simulink model "noise_suppression"  (R2020b)
settings: Solver=FixedStepDiscrete  StartTime=0.0  StopTime=stopTime  RelTol=1e-3
InitFcn:
  | initCallback
StopFcn:
  | stopCallback
values from neighbouring files (symbols this model uses):
  mp = sm_init_avalon_signals(mp)    [sm_callback_init.m]
undefined symbols (not defined in the file or in its folder): config
libraries: hdlsllib x1
settings Model: Creator=Ross  LastModifiedBy=tyler
settings SolverCC: AutoInsertRateTranBlk=on
settings DataIOCC: ReturnWorkspaceOutputs=off
settings OptimizationCC: BlockReduction=off  ConditionallyExecuteInputs=off  DefaultParameterBehavior=Inlined
settings DebuggingCC: SignalInfNanChecking=error  SignalRangeChecking=warning  ReadBeforeWriteMsg=DisableAll  WriteAfterWriteMsg=DisableAll  WriteAfterReadMsg=DisableAll  AlgebraicLoopMsg=error  MultiTaskDSMMsg=none  SingleTaskRateTransMsg=error  ParameterUnderflowMsg=warning  UnderSpecifiedDataTypeMsg=error  PregeneratedLibrarySubsystemCodeDiagnostic=none  ArithmeticOperatorsInVariantConditions=warning
settings HardwareCC: ProdBitPerPointer=32  ProdBitPerSizeT=32  ProdBitPerPtrDiffT=32  ProdLargestAtomicFloat=None  ProdIntDivRoundTo=Undefined  ProdEndianess=Unspecified  ProdWordSize=32  ProdHWDeviceType=ASIC/FPGA->ASIC/FPGA  TargetBitPerPointer=64  TargetBitPerSizeT=64  TargetBitPerPtrDiffT=64  TargetLongLongMode=on  TargetIntDivRoundTo=Zero  TargetEndianess=LittleEndian  TargetWordSize=64  TargetHWDeviceType=Custom Processor->MATLAB Host Computer  ProdEqTarget=off
settings ModelReferenceCC: UpdateModelReferenceTargets=IfOutOfDate
settings SFSimCC: SFSimEcho=off  SimUseLocalCustomCode=off  CustomCodeUndefinedFunction=UseInterfaceOnly
settings RTWCC: RTWUseLocalCustomCode=off

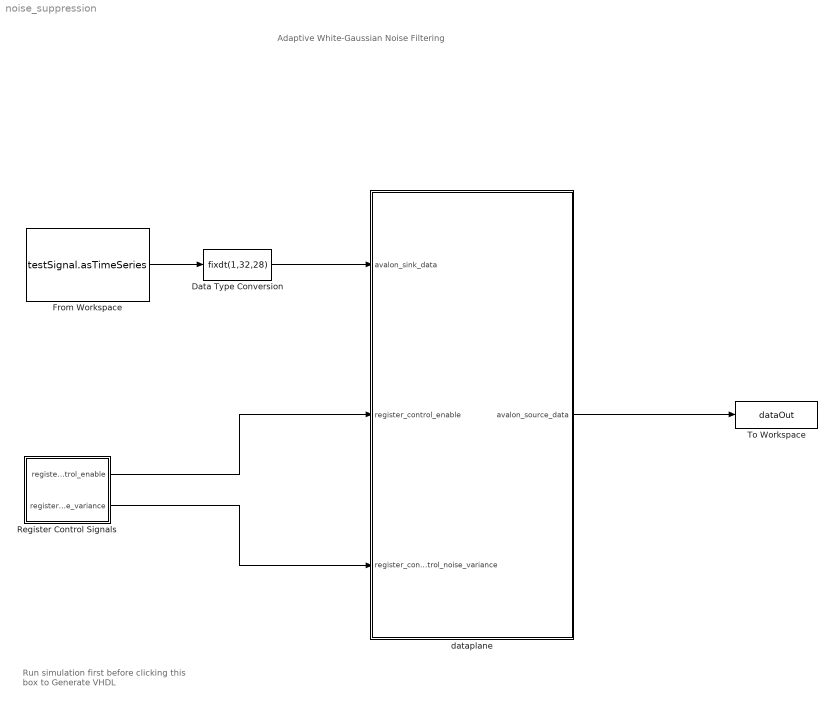
== system noise_suppression ==
  note: Adaptive White-Gaussian Noise Filtering
  note: Run simulation first
      | before clicking this box to
      | Generate VHDL
  Data Type Conversion : DataTypeConversion  OutDataTypeStr=fixdt(1,32,28)
  From Workspace : FromWorkspace  VariableName=testSignal.asTimeSeries  OutDataTypeStr=double  SampleTime=1 / config.system.sampleClockFrequency  Interpolate=off  OutputAfterFinalValue=Setting to zero
  Register Control Signals : Subsystem
  To Workspace : ToWorkspace  VariableName=dataOut  SaveFormat=Timeseries  SampleTime=-1
      settings: Save2DSignal=2-D array (concatenate along first dimension)
  dataplane : Subsystem  TreatAsAtomicUnit=on
  wires:
  dataplane/1(avalon_source_data) -> To Workspace/1
  From Workspace/1 -> Data Type Conversion/1
  Data Type Conversion/1 -> dataplane/1(avalon_sink_data)
  Register Control Signals/1(register_control_enable) -> dataplane/2(register_control_enable)
  Register Control Signals/2(register_control_noise_variance) -> dataplane/3(register_control_noise_variance)

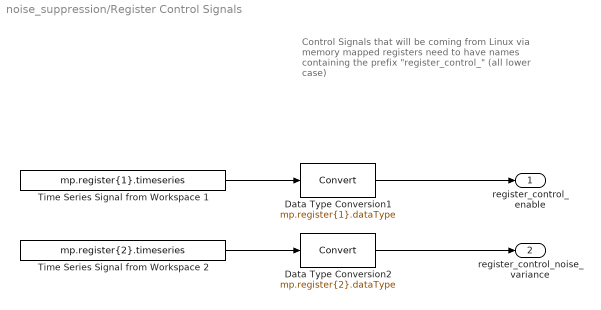
== system noise_suppression/Register Control Signals ==
  note: Control Signals that will be coming from Linux via
      | memory mapped registers need to have names
      | containing the prefix "register_control_"
      | (all lower case)
  Data Type Conversion1 : DataTypeConversion  OutDataTypeStr=mp.register{1}.dataType
  Data Type Conversion2 : DataTypeConversion  OutDataTypeStr=mp.register{2}.dataType
  Time Series Signal from Workspace 1 : FromWorkspace  VariableName=mp.register{1}.timeseries  OutDataTypeStr=double  SampleTime=1 / config.system.sampleClockFrequency
  Time Series Signal from Workspace 2 : FromWorkspace  VariableName=mp.register{2}.timeseries  OutDataTypeStr=double  SampleTime=1 / config.system.sampleClockFrequency
  register_control_enable : Outport  VectorParamsAs1DForOutWhenUnconnected=off
  register_control_noise_variance : Outport  Port=2  VectorParamsAs1DForOutWhenUnconnected=off
  wires:
  Time Series Signal from Workspace 1/1 -> Data Type Conversion1/1
  Data Type Conversion1/1 -> register_control_enable/1
  Time Series Signal from Workspace 2/1 -> Data Type Conversion2/1
  Data Type Conversion2/1 -> register_control_noise_variance/1

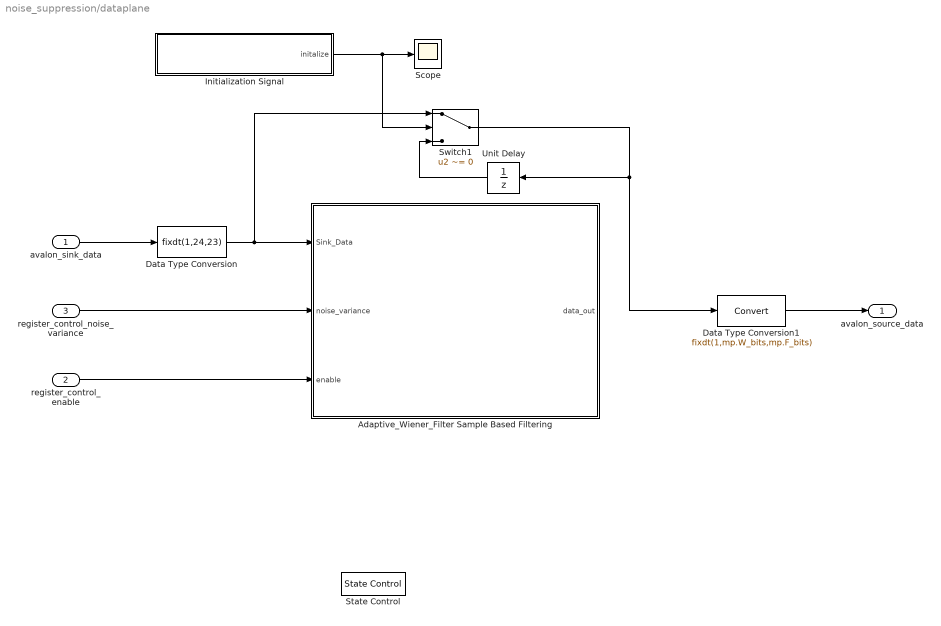
== system noise_suppression/dataplane ==
  avalon_sink_data : Inport
  register_control_enable : Inport  Port=2
  register_control_noise_variance : Inport  Port=3
  Adaptive_Wiener_Filter Sample Based Filtering : Subsystem
  Data Type Conversion : DataTypeConversion  OutDataTypeStr=fixdt(1,24,23)
  Data Type Conversion1 : DataTypeConversion  OutDataTypeStr=fixdt(1,mp.W_bits,mp.F_bits)
  Initialization Signal : Subsystem
  Scope : Scope
  State Control : StateControl  StateControl=Synchronous
  Switch1 : Switch  Criteria=u2 ~= 0  OutDataTypeStr=fixdt(1,24,23)
  Unit Delay : UnitDelay  SampleTime=-1  HasFrameUpgradeWarning=on
  avalon_source_data : Outport  VectorParamsAs1DForOutWhenUnconnected=off
  wires:
  avalon_sink_data/1 -> Data Type Conversion/1
  register_control_enable/1 -> Adaptive_Wiener_Filter Sample Based Filtering/3(enable)
  register_control_noise_variance/1 -> Adaptive_Wiener_Filter Sample Based Filtering/2(noise_variance)
  Data Type Conversion/1 -> Switch1/1, Adaptive_Wiener_Filter Sample Based Filtering/1(Sink_Data)
  Unit Delay/1 -> Switch1/3
  Switch1/1 -> Data Type Conversion1/1, Unit Delay/1
  Data Type Conversion1/1 -> avalon_source_data/1
  Initialization Signal/1(initalize) -> Scope/1, Switch1/2

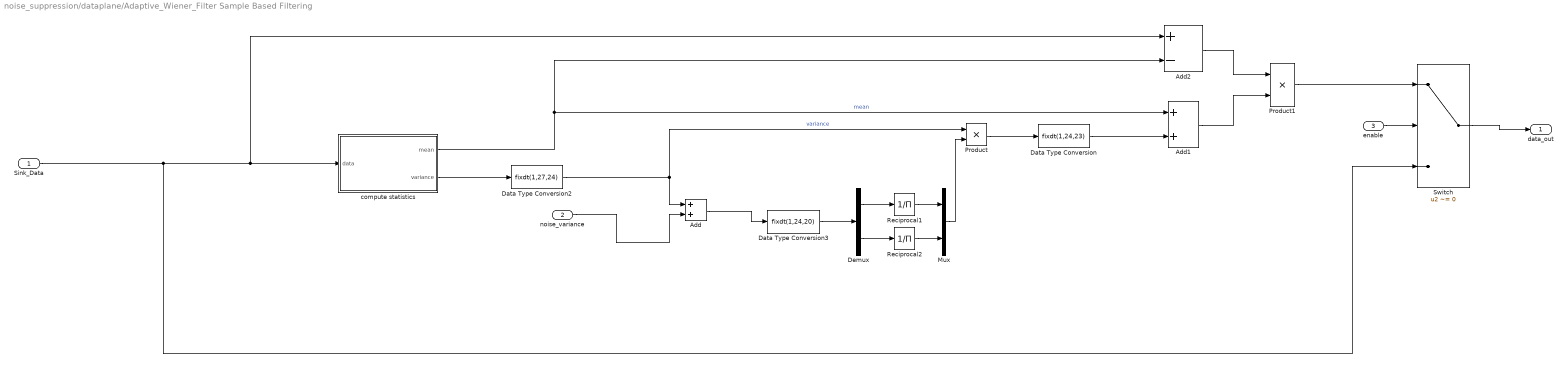
== system noise_suppression/dataplane/Adaptive_Wiener_Filter Sample Based Filtering ==
  Sink_Data : Inport
  noise_variance : Inport  Port=2
  enable : Inport  Port=3
  Add : Sum
  Add1 : Sum
  Add2 : Sum  Inputs=+-
  Data Type Conversion : DataTypeConversion  OutDataTypeStr=fixdt(1,24,23)
  Data Type Conversion2 : DataTypeConversion  OutDataTypeStr=fixdt(1,27,24)
  Data Type Conversion3 : DataTypeConversion  OutDataTypeStr=fixdt(1,24,20)
  Demux : Demux  Outputs=2
  Mux : Mux  Inputs=2
  Product : Product
  Product1 : Product
  Reciprocal1 : Product  Inputs=/  RndMeth=Zero  SaturateOnIntegerOverflow=on
  Reciprocal2 : Product  Inputs=/  RndMeth=Zero  SaturateOnIntegerOverflow=on
  Switch : Switch  Criteria=u2 ~= 0
  compute statistics : Subsystem
  data_out : Outport
  wires:
  compute statistics/1(mean) -> Add2/2, Add1/1  "mean"
  Data Type Conversion/1 -> Add1/2
  Product/1 -> Data Type Conversion/1
  Data Type Conversion2/1 -> Add/1, Product/1  "variance"
  compute statistics/2(variance) -> Data Type Conversion2/1
  Sink_Data/1 -> Switch/3, compute statistics/1(data), Add2/1
  Add2/1 -> Product1/1
  Add1/1 -> Product1/2
  Product1/1 -> Switch/1
  Demux/1 -> Reciprocal1/1
  Demux/2 -> Reciprocal2/1
  Reciprocal2/1 -> Mux/2
  Reciprocal1/1 -> Mux/1
  Switch/1 -> data_out/1
  enable/1 -> Switch/2
  noise_variance/1 -> Add/2
  Add/1 -> Data Type Conversion3/1
  Data Type Conversion3/1 -> Demux/1
  Mux/1 -> Product/2

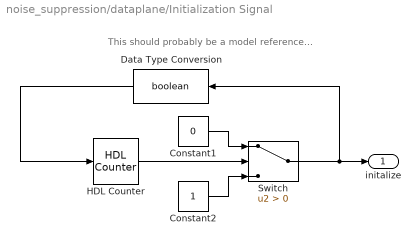
== system noise_suppression/dataplane/Initialization Signal ==
  note: This should probably be a model reference...
  Constant1 : Constant  Value=0
  Constant2 : Constant
  Data Type Conversion : DataTypeConversion  OutDataTypeStr=boolean
  HDL Counter : hdlsllib/Sources/HDL Counter  CountType=Count limited  CountInit=0  CountStep=1  CountMax=2  CountFromType=Initial value  CountFrom=0  CountResetPort=off  CountLoadPort=off  CountEnbPort=on  CountDirPort=off  CountDataType=Unsigned  CountWordLen=2  CountFracLen=0  CountSampTime=-1
  Switch : Switch  Criteria=u2 > Threshold
  initalize : Outport
  wires:
  Constant1/1 -> Switch/1
  Constant2/1 -> Switch/3
  HDL Counter/1 -> Switch/2
  Switch/1 -> Data Type Conversion/1, initalize/1
  Data Type Conversion/1 -> HDL Counter/1

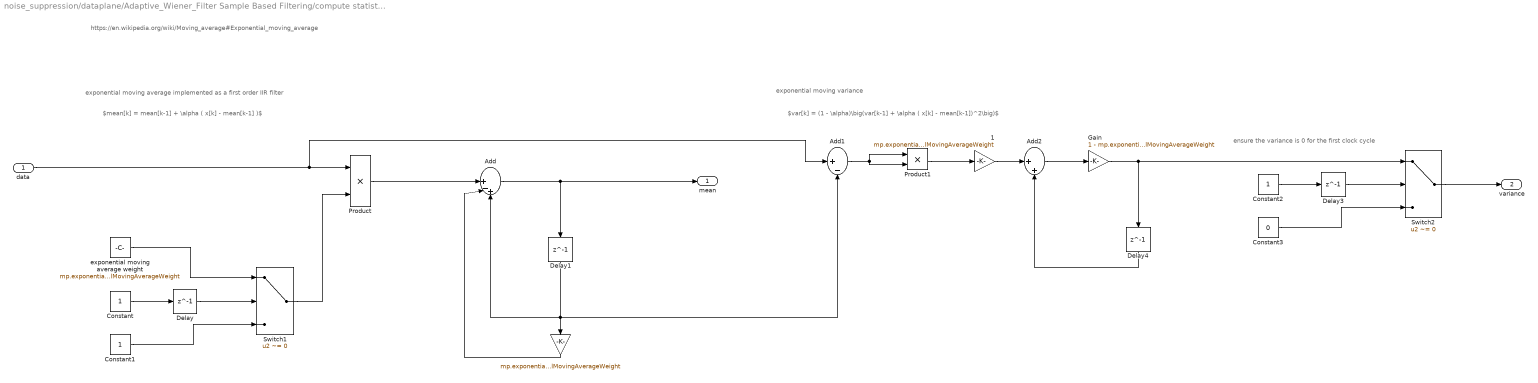
== system noise_suppression/dataplane/Adaptive_Wiener_Filter Sample Based Filtering/compute statistics ==
  note: ensure the variance is 0 for the first clock cycle
  note: https://en.wikipedia.org/wiki/Moving_average#Exponential_moving_average
  note: $mean[k] = mean[k-1] + \alpha ( x[k] - mean[k-1] )$
  note: exponential moving variance
  note: exponential moving average implemented as a first order IIR filter
  note: $var[k] = (1 - \alpha)\big(var[k-1] + \alpha ( x[k] - mean[k-1])^2\big)$
  data : Inport
  " " : Gain  Gain=mp.exponentialMovingAverageWeight  ParamDataTypeStr=Inherit: Inherit from 'Gain'  OutDataTypeStr=Inherit: Inherit via back propagation
  " 1" : Gain  Gain=mp.exponentialMovingAverageWeight  ParamDataTypeStr=Inherit: Inherit from 'Gain'  OutDataTypeStr=Inherit: Same as input
  Add : Sum  Inputs=||+-+  InputSameDT=on  OutDataTypeStr=Inherit: Same as first input
  Add1 : Sum  Inputs=|+-  InputSameDT=on  OutDataTypeStr=Inherit: Same as first input
  Add2 : Sum  Inputs=|++  InputSameDT=on
  Constant : Constant  OutDataTypeStr=boolean  SampleTime=-1
  Constant1 : Constant  OutDataTypeStr=Inherit: Inherit via back propagation  SampleTime=-1
  Constant2 : Constant  OutDataTypeStr=boolean  SampleTime=-1
  Constant3 : Constant  Value=0  OutDataTypeStr=Inherit: Inherit via back propagation  SampleTime=-1
  Delay{,1,3..4} (4 alike) : Delay  DelayLength=1  InitialCondition=0
  Gain : Gain  Gain=1 - mp.exponentialMovingAverageWeight  ParamDataTypeStr=Inherit: Inherit from 'Gain'  OutDataTypeStr=Inherit: Same as input
  Product : Product  OutDataTypeStr=Inherit: Same as first input
  Product1 : Product  OutMin=-2  OutMax=2  OutDataTypeStr=fixdt(1,50)
  Switch1 : Switch  Criteria=u2 ~= 0  InputSameDT=on
  Switch2 : Switch  Criteria=u2 ~= 0  InputSameDT=on
  exponential moving average weight : Constant  Value=mp.exponentialMovingAverageWeight  SampleTime=-1
  mean : Outport  InitialOutput=0
  variance : Outport  Port=2  InitialOutput=0
  wires:
  Constant/1 -> Delay/1
  Switch1/1 -> Product/2
  Add2/1 -> Gain/1
  Add1/1 -> Product1/2, Product1/1
  " "/1 -> Add/2
  Constant1/1 -> Switch1/3
  Delay/1 -> Switch1/2
  Product/1 -> Add/1
  exponential moving average weight/1 -> Switch1/1
  Product1/1 -> " 1"/1
  data/1 -> Add1/1, Product/1
  Constant2/1 -> Delay3/1
  Delay3/1 -> Switch2/2
  Constant3/1 -> Switch2/3
  Switch2/1 -> variance/1
  " 1"/1 -> Add2/1
  Add/1 -> mean/1, Delay1/1
  Delay1/1 -> Add1/2, " "/1, Add/3
  Gain/1 -> Switch2/1, Delay4/1
  Delay4/1 -> Add2/2
